simulink model "PlantaHinf_Real"  (R2016a)
settings: Solver=VariableStepAuto  StartTime=0.0  StopTime=inf  RelTol=1e-3
undefined symbols (not defined in the file or in its folder): K1
libraries: arduino_io_lib x5
settings Model: Creator=Julián  LastModifiedBy=i95sa
settings DataIOCC: LimitDataPoints=on  SaveFormat=Array  SignalLoggingSaveFormat=ModelDataLogs
settings DebuggingCC: SolverPrmCheckMsg=warning  MultiTaskDSMMsg=warning  MultiTaskCondExecSysMsg=none
settings HardwareCC: ProdBitPerPointer=32  ProdLargestAtomicFloat=None  ProdIntDivRoundTo=Undefined  ProdEndianess=Unspecified  ProdWordSize=32  ProdHWDeviceType=32-bit Generic
settings ModelReferenceCC: PropagateSignalLabelsOutOfModel=off
settings ConfigComp: CovModelRefEnable=Off

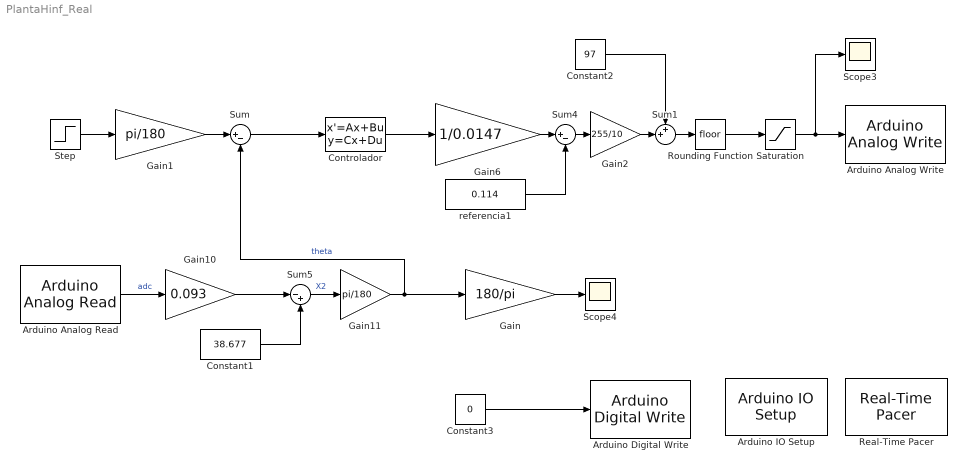
== system PlantaHinf_Real ==
  Arduino Analog Read : arduino_io_lib/Arduino Analog Read  arduinoVar=Existing workspace arduino variable #1  arduinoPin=8  T=0.1
  Arduino Analog Write : arduino_io_lib/Arduino Analog Write  arduinoVar=Existing workspace arduino variable #1  arduinoPin=3  T=0.1
  Arduino Digital Write : arduino_io_lib/Arduino Digital Write  arduinoVar=Existing workspace arduino variable #1  arduinoPin=12  T=0.1
  Arduino IO Setup : arduino_io_lib/Arduino IO Setup  Priority=3  arduinoVar=Existing workspace arduino variable #1  workspaceVarName=ard  comPort=4
  Constant1 : Constant  Value=38.677
  Constant2 : Constant  Value=97
  Constant3 : Constant  Value=0
  Controlador : StateSpace  A=K1.a  B=K1.b  C=K1.c  D=K1.d  X0=0
  Gain : Gain  Gain=180/pi
  Gain1 : Gain  Gain=pi/180
  Gain10 : Gain  Gain=0.093
  Gain11 : Gain  Gain=pi/180
  Gain2 : Gain  Gain=255/10
  Gain6 : Gain  Gain=1/0.0147
  Real-Time Pacer : arduino_io_lib/Real-Time Pacer  simTimePerRealTime=1
  Rounding Function : Rounding
  Saturation : Saturate  UpperLimit=255  LowerLimit=0
  Scope3 : Scope
  Scope4 : Scope
  Step : Step  Time=0  After=0  SampleTime=0
  Sum : Sum  Inputs=|+-
  Sum1 : Sum  Inputs=++|
  Sum4 : Sum  Inputs=|+-
  Sum5 : Sum  Inputs=|-+
  referencia1 : Constant  Value=0.114
  wires:
  Step/1 -> Gain1/1
  Sum/1 -> Controlador/1
  Controlador/1 -> Gain6/1
  Gain/1 -> Scope4/1
  Gain1/1 -> Sum/1
  referencia1/1 -> Sum4/2
  Sum4/1 -> Gain2/1
  Sum1/1 -> Rounding Function/1
  Constant2/1 -> Sum1/1
  Gain2/1 -> Sum1/2
  Gain6/1 -> Sum4/1
  Rounding Function/1 -> Saturation/1
  Arduino Analog Read/1 -> Gain10/1  "adc"
  Gain10/1 -> Sum5/1
  Constant1/1 -> Sum5/2
  Sum5/1 -> Gain11/1  "X2"
  Gain11/1 -> Gain/1, Sum/2  "theta"
  Constant3/1 -> Arduino Digital Write/1
  Saturation/1 -> Scope3/1, Arduino Analog Write/1
